simulink model "Equaliazer"  (R2016a)
settings: Solver=FixedStepDiscrete  SolverMode=SingleTasking  StartTime=0.0  StopTime=inf  RelTol=1e-3
libraries: dspsnks4 x1, dspvision x1
settings Model: Creator=jbarboza  LastModifiedBy=jbarboza
settings SolverCC: AutoInsertRateTranBlk=on
settings DataIOCC: LimitDataPoints=on  SaveOutput=off  SignalLogging=off  SaveTime=off
settings DebuggingCC: AlgebraicLoopMsg=error  SingleTaskRateTransMsg=error  AllowSymbolicDim=off
settings ConfigComp: CovModelRefEnable=Off  CovSFcnEnable=off

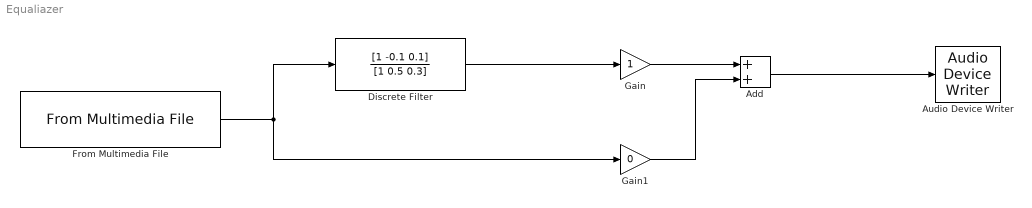
== system Equaliazer ==
  Add : Sum
  Audio Device Writer : dspsnks4/Audio Device Writer  Driver=DirectSound  Device=Default  InheritSampleRate=on  SampleRate=44100  BitDepth=16-bit integer  BufferSize=4096  NumBuffers=10  DefaultOutputChannelMapping=on  OutputChannelMapping=1:2  OutputNumUnderrunSamples=off  DriverIdx=1  DeviceWarnFlag=''
  Discrete Filter : DiscreteFilter  Numerator=[1 -0.1 0.1]  Denominator=[1 0.5 0.3]
  From Multimedia File : dspvision/From Multimedia File  inputFilename=C:\Users\jbarboza\Documents\Cursos\I Semestre 2017\Procesamiento Digital de Señales EL-5805\MediaPlayer\The Cranberries - Zombie.wav  loop=on  numPlays=inf  outputStreams=Audio only  videoDataType=single  audioDataType=double  inheritSampleTime=on  userDefinedSampleTime=1/30  noAudioOutput=off  isIntensityVideo=off  fourcc=RGB  colorVideoFormat=Separate color signals  outputEOF=off  dataOrg=Column-major  audioFrameSize=1024  computeAudioFrameSize=off  outSamplingMode=Sample based
  Gain : Gain
  Gain1 : Gain  Gain=0
  wires:
  Gain/1 -> Add/1
  Gain1/1 -> Add/2
  Add/1 -> Audio Device Writer/1
  Discrete Filter/1 -> Gain/1
  From Multimedia File/1 -> Gain1/1, Discrete Filter/1
